simulink model "sim01"  (R2020a)
settings: Solver=VariableStepAuto  StartTime=0.0  StopTime=1000.0  MaxStep=2  RelTol=1e-3
values from neighbouring files (symbols this model uses):
  dt = 1    [skrypt01.m]
  k = 15    [skrypt01.m]
  M = [T,1]    [skrypt01.m]
  T0 = 30    [skrypt01.m]
settings Model: Creator=jakub  LastModifiedBy=jakub

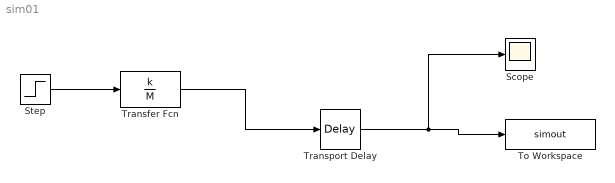
== system sim01 ==
  Scope : Scope
  Step : Step  Time=0  After=dt  SampleTime=0
  To Workspace : ToWorkspace  VariableName=simout  SampleTime=-1
  Transfer Fcn : TransferFcn  Numerator=k  Denominator=M
  Transport Delay : TransportDelay  DelayTime=T0
  wires:
  Step/1 -> Transfer Fcn/1
  Transport Delay/1 -> Scope/1, To Workspace/1
  Transfer Fcn/1 -> Transport Delay/1
